simulink model "falcon9"  (R2020a)
settings: Solver=VariableStepAuto  StartTime=0.0  StopTime=100  RelTol=1e-3
values from neighbouring files (symbols this model uses):
  alpha = 5e-4    (= 0.0005)    [init.m]
  dt = tf/N2    [cvx_solve.m]    (also in init.m = 0.5)
  g = [-3.71,0,0]'    [init.m]
  N2 = 80    [init.m]
undefined symbols (not defined in the file or in its folder): Earth, WGS84, x, z
libraries: aerolibtransform2 x1, aerolibfltsims x1, shared6dof x1
settings Model: Creator=robin  LastModifiedBy=robin

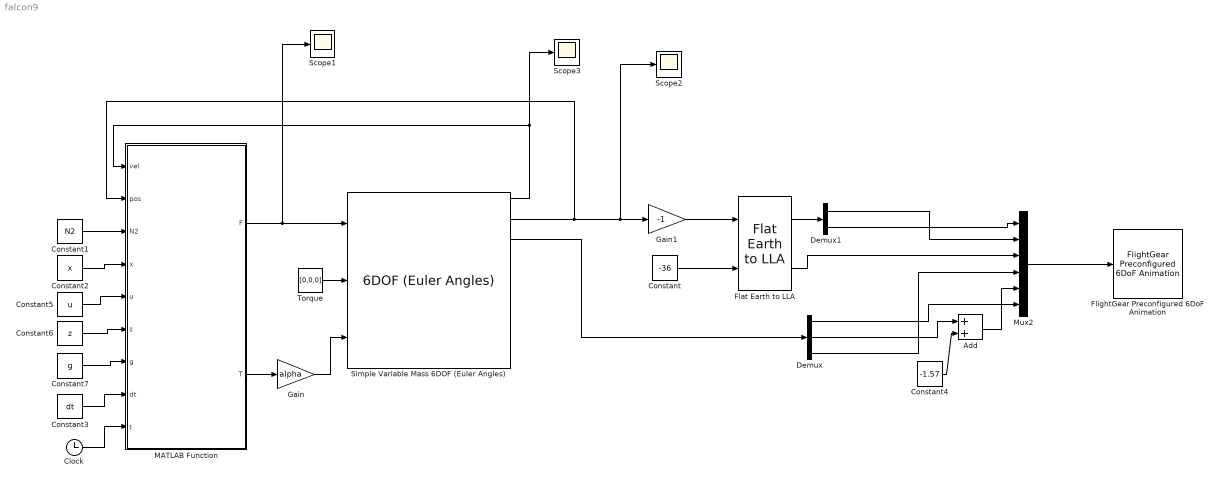
== system falcon9 ==
  Add : Sum
  Clock : Clock
  Constant : Constant  Value=-36
  Constant1 : Constant  Value=N2
  Constant2 : Constant  Value=x
  Constant3 : Constant  Value=dt
  Constant4 : Constant  Value=-1.57
  Constant5 : Constant  Value=u
  Constant6 : Constant  Value=z
  Constant7 : Constant  Value=g
  Demux : Demux  Outputs=3
  Demux1 : Demux  Outputs=2
  Flat Earth to LLA : aerolibtransform2/Flat Earth to LLA  units=Metric (MKS)  ptype=Earth (WGS84)  F=1/298.257223563  R=6378137  refPosPort=off  LL0=[21.3139 -157.927]  psi=0
  FlightGear Preconfigured 6DoF Animation : aerolibfltsims/FlightGear Preconfigured 6DoF Animation  xFlightGearVersion=v2019.1  DestinationIpAddress=127.0.0.1  DestinationPort=5502  SampleTime=1/150  packetVersion=24
  Gain : Gain  Gain=alpha
  Gain1 : Gain  Gain=-1
  MATLAB Function : MATLAB Function  TreatAsAtomicUnit=on
  Mux2 : Mux  Inputs=6
  Scope1 : Scope
  Scope2 : Scope
  Scope3 : Scope
  Simple Variable Mass 6DOF (Euler Angles) : shared6dof/6DOF (Euler Angles)  units=Metric (MKS)  mtype=Simple Variable  rep=Euler Angles  xme_0=[450,-330,2400]  Vm_0=[0 0 0]  eul_0=[0 1.57 0]  pm_0=[0 0 0]  mass_0=2e3  mass_e=1.7e3  mass_f=2e3  inertia=eye(3)  inertia_e=eye(3)  inertia_f=2*eye(3)  k_quat=1.0  vre_flag=off  abi_flag=off  aMode=0  xme_statename=''  Vm_statename=''  eul_statename=''  quat_statename=''  pm_statename=''  mass_statename=''
      settings: SourceProductBaseCode=AE,PW,MT,VE,VP
  Torque : Constant  Value=[0,0,0]
  wires:
  Constant/1 -> Flat Earth to LLA/2
  Simple Variable Mass 6DOF (Euler Angles)/3 -> Demux/1
  Demux/3 -> Mux2/4
  Flat Earth to LLA/1 -> Demux1/1
  Flat Earth to LLA/2 -> Mux2/3
  Mux2/1 -> FlightGear Preconfigured 6DoF Animation/1
  Demux/2 -> Add/1
  Add/1 -> Mux2/5
  Constant4/1 -> Add/2
  Demux1/2 -> Mux2/1
  Demux1/1 -> Mux2/2
  Demux/1 -> Mux2/6
  Torque/1 -> Simple Variable Mass 6DOF (Euler Angles)/2
  Simple Variable Mass 6DOF (Euler Angles)/1 -> MATLAB Function/1(vel), Scope3/1
  Constant1/1 -> MATLAB Function/3(N2)
  Constant2/1 -> MATLAB Function/4(x)
  Constant5/1 -> MATLAB Function/5(u)
  Constant6/1 -> MATLAB Function/6(z)
  Constant7/1 -> MATLAB Function/7(g)
  MATLAB Function/1(F) -> Scope1/1, Simple Variable Mass 6DOF (Euler Angles)/1
  Gain/1 -> Simple Variable Mass 6DOF (Euler Angles)/3
  MATLAB Function/2(T) -> Gain/1
  Simple Variable Mass 6DOF (Euler Angles)/2 -> MATLAB Function/2(pos), Scope2/1, Gain1/1
  Constant3/1 -> MATLAB Function/8(dt)
  Clock/1 -> MATLAB Function/9(t)
  Gain1/1 -> Flat Earth to LLA/1

== matlab function falcon9/MATLAB Function ==
  settings: updateMethod=DISCRETE
  data: vel input; pos input; F output; N2 input; x input; u input; z input; g input; T output; dt input; t input
function [F,T]= guidance(vel,pos,N2,x,u,z,g,dt,t)
    pos = [pos(3);pos(1);pos(2)];
    vel = [vel(3);vel(1);vel(2)];
    step = ceil((t+1e-6)/dt);
    Kx = 0.5;
    Kv = 0.8;
%     figure(1)
%     hold on
    if step <N2
        m = exp(z(step));
        thrust = Kx*m*(x(1:3,step+1)-pos)+u(:,step+1)*m+Kv*m*(0.5*(x(4:6,step+1)+x(4:6,step))-vel);
        T = norm(thrust);
        F = thrust + m*g;
        F = [-F(1);F(3);F(2)];
    else
        F=[0;0;0];
        T=0;
    end
%     plot(x(3,step+1),x(1,step+1),'o');
%     plot(pos(3),pos(1),'.')
%     if norm(pos-x(1:3,step+1))<5
%         step = step+1;
%     end
end
